simulink model "r2_deng_tvg_rev1_13"  (R2012b)
settings: Solver=VariableStepDiscrete  StartTime=0.0  StopTime=2000  RelTol=1e-3
libraries: xbsIndex_r4 x7993, casper_library_misc x17, casper_library_sources x12, casper_library_communications x4, simulink x3, xps_library x2
(part 9 of 65)

== system r2_deng_tvg_rev1_13/bus_expand3 ==
  bus_in : Inport
  gatewayOut{1..8} (8 alike) : xbsIndex_r4/Gateway Out  inherit_from_input=off  hdl_port=off  timing_constraint=None  locs_specified=off  LOCs={}  UseAsDAC=off  DACChannel='1'  block_type=gatewayout
  reinterpret{1..8} (8 alike) : xbsIndex_r4/Reinterpret  force_arith_type=on  arith_type="Signed  (2's comp)"  force_bin_pt=on  bin_pt=19  block_type=reinterpret
  slice1 : xbsIndex_r4/Slice  nbits=20  boolean_output=off  mode=Upper Bit Location + Width  bit1=-140  base1=MSB of Input  bit0=0  base0=LSB of Input  dbl_ovrd=off  block_type=slice
  slice2 : xbsIndex_r4/Slice  nbits=20  boolean_output=off  mode=Upper Bit Location + Width  bit1=-120  base1=MSB of Input  bit0=0  base0=LSB of Input  dbl_ovrd=off  block_type=slice
  slice3 : xbsIndex_r4/Slice  nbits=20  boolean_output=off  mode=Upper Bit Location + Width  bit1=-100  base1=MSB of Input  bit0=0  base0=LSB of Input  dbl_ovrd=off  block_type=slice
  slice4 : xbsIndex_r4/Slice  nbits=20  boolean_output=off  mode=Upper Bit Location + Width  bit1=-80  base1=MSB of Input  bit0=0  base0=LSB of Input  dbl_ovrd=off  block_type=slice
  slice5 : xbsIndex_r4/Slice  nbits=20  boolean_output=off  mode=Upper Bit Location + Width  bit1=-60  base1=MSB of Input  bit0=0  base0=LSB of Input  dbl_ovrd=off  block_type=slice
  slice6 : xbsIndex_r4/Slice  nbits=20  boolean_output=off  mode=Upper Bit Location + Width  bit1=-40  base1=MSB of Input  bit0=0  base0=LSB of Input  dbl_ovrd=off  block_type=slice
  slice7 : xbsIndex_r4/Slice  nbits=20  boolean_output=off  mode=Upper Bit Location + Width  bit1=-20  base1=MSB of Input  bit0=0  base0=LSB of Input  dbl_ovrd=off  block_type=slice
  slice8 : xbsIndex_r4/Slice  nbits=20  boolean_output=off  mode=Upper Bit Location + Width  bit1=0  base1=MSB of Input  bit0=0  base0=LSB of Input  dbl_ovrd=off  block_type=slice
  toWorkspace1 : ToWorkspace  VariableName=wng0_tp0_1  SampleTime=-1  SaveFormat=Structure With Time
  toWorkspace2 : ToWorkspace  VariableName=wng0_tp0_2  SampleTime=-1  SaveFormat=Structure With Time
  toWorkspace3 : ToWorkspace  VariableName=wng0_tp0_3  SampleTime=-1  SaveFormat=Structure With Time
  toWorkspace4 : ToWorkspace  VariableName=wng0_tp0_4  SampleTime=-1  SaveFormat=Structure With Time
  toWorkspace5 : ToWorkspace  VariableName=wng0_tp0_5  SampleTime=-1  SaveFormat=Structure With Time
  toWorkspace6 : ToWorkspace  VariableName=wng0_tp0_6  SampleTime=-1  SaveFormat=Structure With Time
  toWorkspace7 : ToWorkspace  VariableName=wng0_tp0_7  SampleTime=-1  SaveFormat=Structure With Time
  toWorkspace8 : ToWorkspace  VariableName=wng0_tp0_8  SampleTime=-1  SaveFormat=Structure With Time
  msb_out8 : Outport
  out7 : Outport  Port=2
  out6 : Outport  Port=3
  out5 : Outport  Port=4
  out4 : Outport  Port=5
  out3 : Outport  Port=6
  out2 : Outport  Port=7
  lsb_out1 : Outport  Port=8
  wires:
  bus_in/1 -> slice8/1, slice7/1, slice6/1, slice5/1, slice4/1, slice3/1, slice2/1, slice1/1
  slice8/1 -> reinterpret8/1
  reinterpret8/1 -> gatewayOut8/1, msb_out8/1
  gatewayOut8/1 -> toWorkspace8/1
  slice7/1 -> reinterpret7/1
  reinterpret7/1 -> gatewayOut7/1, out7/1
  gatewayOut7/1 -> toWorkspace7/1
  slice6/1 -> reinterpret6/1
  reinterpret6/1 -> gatewayOut6/1, out6/1
  gatewayOut6/1 -> toWorkspace6/1
  slice5/1 -> reinterpret5/1
  reinterpret5/1 -> gatewayOut5/1, out5/1
  gatewayOut5/1 -> toWorkspace5/1
  slice4/1 -> reinterpret4/1
  reinterpret4/1 -> gatewayOut4/1, out4/1
  gatewayOut4/1 -> toWorkspace4/1
  slice3/1 -> reinterpret3/1
  reinterpret3/1 -> gatewayOut3/1, out3/1
  gatewayOut3/1 -> toWorkspace3/1
  slice2/1 -> reinterpret2/1
  reinterpret2/1 -> gatewayOut2/1, out2/1
  gatewayOut2/1 -> toWorkspace2/1
  slice1/1 -> reinterpret1/1
  reinterpret1/1 -> gatewayOut1/1, lsb_out1/1
  gatewayOut1/1 -> toWorkspace1/1

== system r2_deng_tvg_rev1_13/bus_expand4 ==
  bus_in : Inport
  gatewayOut{1..8} (8 alike) : xbsIndex_r4/Gateway Out  inherit_from_input=off  hdl_port=off  timing_constraint=None  locs_specified=off  LOCs={}  UseAsDAC=off  DACChannel='1'  block_type=gatewayout
  reinterpret{1..8} (8 alike) : xbsIndex_r4/Reinterpret  force_arith_type=on  arith_type="Signed  (2's comp)"  force_bin_pt=on  bin_pt=17  block_type=reinterpret
  slice1 : xbsIndex_r4/Slice  nbits=18  boolean_output=off  mode=Upper Bit Location + Width  bit1=-126  base1=MSB of Input  bit0=0  base0=LSB of Input  dbl_ovrd=off  block_type=slice
  slice2 : xbsIndex_r4/Slice  nbits=18  boolean_output=off  mode=Upper Bit Location + Width  bit1=-108  base1=MSB of Input  bit0=0  base0=LSB of Input  dbl_ovrd=off  block_type=slice
  slice3 : xbsIndex_r4/Slice  nbits=18  boolean_output=off  mode=Upper Bit Location + Width  bit1=-90  base1=MSB of Input  bit0=0  base0=LSB of Input  dbl_ovrd=off  block_type=slice
  slice4 : xbsIndex_r4/Slice  nbits=18  boolean_output=off  mode=Upper Bit Location + Width  bit1=-72  base1=MSB of Input  bit0=0  base0=LSB of Input  dbl_ovrd=off  block_type=slice
  slice5 : xbsIndex_r4/Slice  nbits=18  boolean_output=off  mode=Upper Bit Location + Width  bit1=-54  base1=MSB of Input  bit0=0  base0=LSB of Input  dbl_ovrd=off  block_type=slice
  slice6 : xbsIndex_r4/Slice  nbits=18  boolean_output=off  mode=Upper Bit Location + Width  bit1=-36  base1=MSB of Input  bit0=0  base0=LSB of Input  dbl_ovrd=off  block_type=slice
  slice7 : xbsIndex_r4/Slice  nbits=18  boolean_output=off  mode=Upper Bit Location + Width  bit1=-18  base1=MSB of Input  bit0=0  base0=LSB of Input  dbl_ovrd=off  block_type=slice
  slice8 : xbsIndex_r4/Slice  nbits=18  boolean_output=off  mode=Upper Bit Location + Width  bit1=0  base1=MSB of Input  bit0=0  base0=LSB of Input  dbl_ovrd=off  block_type=slice
  toWorkspace1 : ToWorkspace  VariableName=cwg1_tp0_1  SampleTime=-1  SaveFormat=Structure With Time
  toWorkspace2 : ToWorkspace  VariableName=cwg1_tp0_2  SampleTime=-1  SaveFormat=Structure With Time
  toWorkspace3 : ToWorkspace  VariableName=cwg1_tp0_3  SampleTime=-1  SaveFormat=Structure With Time
  toWorkspace4 : ToWorkspace  VariableName=cwg1_tp0_4  SampleTime=-1  SaveFormat=Structure With Time
  toWorkspace5 : ToWorkspace  VariableName=cwg1_tp0_5  SampleTime=-1  SaveFormat=Structure With Time
  toWorkspace6 : ToWorkspace  VariableName=cwg1_tp0_6  SampleTime=-1  SaveFormat=Structure With Time
  toWorkspace7 : ToWorkspace  VariableName=cwg1_tp0_7  SampleTime=-1  SaveFormat=Structure With Time
  toWorkspace8 : ToWorkspace  VariableName=cwg1_tp0_8  SampleTime=-1  SaveFormat=Structure With Time
  msb_out8 : Outport
  out7 : Outport  Port=2
  out6 : Outport  Port=3
  out5 : Outport  Port=4
  out4 : Outport  Port=5
  out3 : Outport  Port=6
  out2 : Outport  Port=7
  lsb_out1 : Outport  Port=8
  wires:
  bus_in/1 -> slice8/1, slice7/1, slice6/1, slice5/1, slice4/1, slice3/1, slice2/1, slice1/1
  slice8/1 -> reinterpret8/1
  reinterpret8/1 -> gatewayOut8/1, msb_out8/1
  gatewayOut8/1 -> toWorkspace8/1
  slice7/1 -> reinterpret7/1
  reinterpret7/1 -> gatewayOut7/1, out7/1
  gatewayOut7/1 -> toWorkspace7/1
  slice6/1 -> reinterpret6/1
  reinterpret6/1 -> gatewayOut6/1, out6/1
  gatewayOut6/1 -> toWorkspace6/1
  slice5/1 -> reinterpret5/1
  reinterpret5/1 -> gatewayOut5/1, out5/1
  gatewayOut5/1 -> toWorkspace5/1
  slice4/1 -> reinterpret4/1
  reinterpret4/1 -> gatewayOut4/1, out4/1
  gatewayOut4/1 -> toWorkspace4/1
  slice3/1 -> reinterpret3/1
  reinterpret3/1 -> gatewayOut3/1, out3/1
  gatewayOut3/1 -> toWorkspace3/1
  slice2/1 -> reinterpret2/1
  reinterpret2/1 -> gatewayOut2/1, out2/1
  gatewayOut2/1 -> toWorkspace2/1
  slice1/1 -> reinterpret1/1
  reinterpret1/1 -> gatewayOut1/1, lsb_out1/1
  gatewayOut1/1 -> toWorkspace1/1

== system r2_deng_tvg_rev1_13/bus_expand6 ==
  bus_in : Inport
  gatewayOut{1..8} (8 alike) : xbsIndex_r4/Gateway Out  inherit_from_input=off  hdl_port=off  timing_constraint=None  locs_specified=off  LOCs={}  UseAsDAC=off  DACChannel='1'  block_type=gatewayout
  reinterpret{1..8} (8 alike) : xbsIndex_r4/Reinterpret  force_arith_type=on  arith_type="Signed  (2's comp)"  force_bin_pt=on  bin_pt=9  block_type=reinterpret
  slice1 : xbsIndex_r4/Slice  nbits=10  boolean_output=off  mode=Upper Bit Location + Width  bit1=-70  base1=MSB of Input  bit0=0  base0=LSB of Input  dbl_ovrd=off  block_type=slice
  slice2 : xbsIndex_r4/Slice  nbits=10  boolean_output=off  mode=Upper Bit Location + Width  bit1=-60  base1=MSB of Input  bit0=0  base0=LSB of Input  dbl_ovrd=off  block_type=slice
  slice3 : xbsIndex_r4/Slice  nbits=10  boolean_output=off  mode=Upper Bit Location + Width  bit1=-50  base1=MSB of Input  bit0=0  base0=LSB of Input  dbl_ovrd=off  block_type=slice
  slice4 : xbsIndex_r4/Slice  nbits=10  boolean_output=off  mode=Upper Bit Location + Width  bit1=-40  base1=MSB of Input  bit0=0  base0=LSB of Input  dbl_ovrd=off  block_type=slice
  slice5 : xbsIndex_r4/Slice  nbits=10  boolean_output=off  mode=Upper Bit Location + Width  bit1=-30  base1=MSB of Input  bit0=0  base0=LSB of Input  dbl_ovrd=off  block_type=slice
  slice6 : xbsIndex_r4/Slice  nbits=10  boolean_output=off  mode=Upper Bit Location + Width  bit1=-20  base1=MSB of Input  bit0=0  base0=LSB of Input  dbl_ovrd=off  block_type=slice
  slice7 : xbsIndex_r4/Slice  nbits=10  boolean_output=off  mode=Upper Bit Location + Width  bit1=-10  base1=MSB of Input  bit0=0  base0=LSB of Input  dbl_ovrd=off  block_type=slice
  slice8 : xbsIndex_r4/Slice  nbits=10  boolean_output=off  mode=Upper Bit Location + Width  bit1=0  base1=MSB of Input  bit0=0  base0=LSB of Input  dbl_ovrd=off  block_type=slice
  toWorkspace1 : ToWorkspace  VariableName=cwg1_tp2_1  SampleTime=-1  SaveFormat=Structure With Time
  toWorkspace2 : ToWorkspace  VariableName=cwg1_tp2_2  SampleTime=-1  SaveFormat=Structure With Time
  toWorkspace3 : ToWorkspace  VariableName=cwg1_tp2_3  SampleTime=-1  SaveFormat=Structure With Time
  toWorkspace4 : ToWorkspace  VariableName=cwg1_tp2_4  SampleTime=-1  SaveFormat=Structure With Time
  toWorkspace5 : ToWorkspace  VariableName=cwg1_tp2_5  SampleTime=-1  SaveFormat=Structure With Time
  toWorkspace6 : ToWorkspace  VariableName=cwg1_tp2_6  SampleTime=-1  SaveFormat=Structure With Time
  toWorkspace7 : ToWorkspace  VariableName=cwg1_tp2_7  SampleTime=-1  SaveFormat=Structure With Time
  toWorkspace8 : ToWorkspace  VariableName=cwg1_tp2_8  SampleTime=-1  SaveFormat=Structure With Time
  msb_out8 : Outport
  out7 : Outport  Port=2
  out6 : Outport  Port=3
  out5 : Outport  Port=4
  out4 : Outport  Port=5
  out3 : Outport  Port=6
  out2 : Outport  Port=7
  lsb_out1 : Outport  Port=8
  wires:
  bus_in/1 -> slice8/1, slice7/1, slice6/1, slice5/1, slice4/1, slice3/1, slice2/1, slice1/1
  slice8/1 -> reinterpret8/1
  reinterpret8/1 -> gatewayOut8/1, msb_out8/1
  gatewayOut8/1 -> toWorkspace8/1
  slice7/1 -> reinterpret7/1
  reinterpret7/1 -> gatewayOut7/1, out7/1
  gatewayOut7/1 -> toWorkspace7/1
  slice6/1 -> reinterpret6/1
  reinterpret6/1 -> gatewayOut6/1, out6/1
  gatewayOut6/1 -> toWorkspace6/1
  slice5/1 -> reinterpret5/1
  reinterpret5/1 -> gatewayOut5/1, out5/1
  gatewayOut5/1 -> toWorkspace5/1
  slice4/1 -> reinterpret4/1
  reinterpret4/1 -> gatewayOut4/1, out4/1
  gatewayOut4/1 -> toWorkspace4/1
  slice3/1 -> reinterpret3/1
  reinterpret3/1 -> gatewayOut3/1, out3/1
  gatewayOut3/1 -> toWorkspace3/1
  slice2/1 -> reinterpret2/1
  reinterpret2/1 -> gatewayOut2/1, out2/1
  gatewayOut2/1 -> toWorkspace2/1
  slice1/1 -> reinterpret1/1
  reinterpret1/1 -> gatewayOut1/1, lsb_out1/1
  gatewayOut1/1 -> toWorkspace1/1

== system r2_deng_tvg_rev1_13/bus_expand8 ==
  bus_in : Inport
  gatewayOut{1..8} (8 alike) : xbsIndex_r4/Gateway Out  inherit_from_input=off  hdl_port=off  timing_constraint=None  locs_specified=off  LOCs={}  UseAsDAC=off  DACChannel='1'  block_type=gatewayout
  reinterpret{1..8} (8 alike) : xbsIndex_r4/Reinterpret  force_arith_type=on  arith_type="Signed  (2's comp)"  force_bin_pt=on  bin_pt=17  block_type=reinterpret
  slice1 : xbsIndex_r4/Slice  nbits=18  boolean_output=off  mode=Upper Bit Location + Width  bit1=-126  base1=MSB of Input  bit0=0  base0=LSB of Input  dbl_ovrd=off  block_type=slice
  slice2 : xbsIndex_r4/Slice  nbits=18  boolean_output=off  mode=Upper Bit Location + Width  bit1=-108  base1=MSB of Input  bit0=0  base0=LSB of Input  dbl_ovrd=off  block_type=slice
  slice3 : xbsIndex_r4/Slice  nbits=18  boolean_output=off  mode=Upper Bit Location + Width  bit1=-90  base1=MSB of Input  bit0=0  base0=LSB of Input  dbl_ovrd=off  block_type=slice
  slice4 : xbsIndex_r4/Slice  nbits=18  boolean_output=off  mode=Upper Bit Location + Width  bit1=-72  base1=MSB of Input  bit0=0  base0=LSB of Input  dbl_ovrd=off  block_type=slice
  slice5 : xbsIndex_r4/Slice  nbits=18  boolean_output=off  mode=Upper Bit Location + Width  bit1=-54  base1=MSB of Input  bit0=0  base0=LSB of Input  dbl_ovrd=off  block_type=slice
  slice6 : xbsIndex_r4/Slice  nbits=18  boolean_output=off  mode=Upper Bit Location + Width  bit1=-36  base1=MSB of Input  bit0=0  base0=LSB of Input  dbl_ovrd=off  block_type=slice
  slice7 : xbsIndex_r4/Slice  nbits=18  boolean_output=off  mode=Upper Bit Location + Width  bit1=-18  base1=MSB of Input  bit0=0  base0=LSB of Input  dbl_ovrd=off  block_type=slice
  slice8 : xbsIndex_r4/Slice  nbits=18  boolean_output=off  mode=Upper Bit Location + Width  bit1=0  base1=MSB of Input  bit0=0  base0=LSB of Input  dbl_ovrd=off  block_type=slice
  toWorkspace1 : ToWorkspace  VariableName=wng1_tp0_1  SampleTime=-1  SaveFormat=Structure With Time
  toWorkspace2 : ToWorkspace  VariableName=wng1_tp0_2  SampleTime=-1  SaveFormat=Structure With Time
  toWorkspace3 : ToWorkspace  VariableName=wng1_tp0_3  SampleTime=-1  SaveFormat=Structure With Time
  toWorkspace4 : ToWorkspace  VariableName=wng1_tp0_4  SampleTime=-1  SaveFormat=Structure With Time
  toWorkspace5 : ToWorkspace  VariableName=wng1_tp0_5  SampleTime=-1  SaveFormat=Structure With Time
  toWorkspace6 : ToWorkspace  VariableName=wng1_tp0_6  SampleTime=-1  SaveFormat=Structure With Time
  toWorkspace7 : ToWorkspace  VariableName=wng1_tp0_7  SampleTime=-1  SaveFormat=Structure With Time
  toWorkspace8 : ToWorkspace  VariableName=wng1_tp0_8  SampleTime=-1  SaveFormat=Structure With Time
  msb_out8 : Outport
  out7 : Outport  Port=2
  out6 : Outport  Port=3
  out5 : Outport  Port=4
  out4 : Outport  Port=5
  out3 : Outport  Port=6
  out2 : Outport  Port=7
  lsb_out1 : Outport  Port=8
  wires:
  bus_in/1 -> slice8/1, slice7/1, slice6/1, slice5/1, slice4/1, slice3/1, slice2/1, slice1/1
  slice8/1 -> reinterpret8/1
  reinterpret8/1 -> gatewayOut8/1, msb_out8/1
  gatewayOut8/1 -> toWorkspace8/1
  slice7/1 -> reinterpret7/1
  reinterpret7/1 -> gatewayOut7/1, out7/1
  gatewayOut7/1 -> toWorkspace7/1
  slice6/1 -> reinterpret6/1
  reinterpret6/1 -> gatewayOut6/1, out6/1
  gatewayOut6/1 -> toWorkspace6/1
  slice5/1 -> reinterpret5/1
  reinterpret5/1 -> gatewayOut5/1, out5/1
  gatewayOut5/1 -> toWorkspace5/1
  slice4/1 -> reinterpret4/1
  reinterpret4/1 -> gatewayOut4/1, out4/1
  gatewayOut4/1 -> toWorkspace4/1
  slice3/1 -> reinterpret3/1
  reinterpret3/1 -> gatewayOut3/1, out3/1
  gatewayOut3/1 -> toWorkspace3/1
  slice2/1 -> reinterpret2/1
  reinterpret2/1 -> gatewayOut2/1, out2/1
  gatewayOut2/1 -> toWorkspace2/1
  slice1/1 -> reinterpret1/1
  reinterpret1/1 -> gatewayOut1/1, lsb_out1/1
  gatewayOut1/1 -> toWorkspace1/1

== system r2_deng_tvg_rev1_13/bus_expand9 ==
  bus_in : Inport
  gatewayOut{1..8} (8 alike) : xbsIndex_r4/Gateway Out  inherit_from_input=off  hdl_port=off  timing_constraint=None  locs_specified=off  LOCs={}  UseAsDAC=off  DACChannel='1'  block_type=gatewayout
  reinterpret{1..8} (8 alike) : xbsIndex_r4/Reinterpret  force_arith_type=on  arith_type=Unsigned  force_bin_pt=on  bin_pt=0  block_type=reinterpret
  slice1 : xbsIndex_r4/Slice  nbits=10  boolean_output=off  mode=Upper Bit Location + Width  bit1=-70  base1=MSB of Input  bit0=0  base0=LSB of Input  dbl_ovrd=off  block_type=slice
  slice2 : xbsIndex_r4/Slice  nbits=10  boolean_output=off  mode=Upper Bit Location + Width  bit1=-60  base1=MSB of Input  bit0=0  base0=LSB of Input  dbl_ovrd=off  block_type=slice
  slice3 : xbsIndex_r4/Slice  nbits=10  boolean_output=off  mode=Upper Bit Location + Width  bit1=-50  base1=MSB of Input  bit0=0  base0=LSB of Input  dbl_ovrd=off  block_type=slice
  slice4 : xbsIndex_r4/Slice  nbits=10  boolean_output=off  mode=Upper Bit Location + Width  bit1=-40  base1=MSB of Input  bit0=0  base0=LSB of Input  dbl_ovrd=off  block_type=slice
  slice5 : xbsIndex_r4/Slice  nbits=10  boolean_output=off  mode=Upper Bit Location + Width  bit1=-30  base1=MSB of Input  bit0=0  base0=LSB of Input  dbl_ovrd=off  block_type=slice
  slice6 : xbsIndex_r4/Slice  nbits=10  boolean_output=off  mode=Upper Bit Location + Width  bit1=-20  base1=MSB of Input  bit0=0  base0=LSB of Input  dbl_ovrd=off  block_type=slice
  slice7 : xbsIndex_r4/Slice  nbits=10  boolean_output=off  mode=Upper Bit Location + Width  bit1=-10  base1=MSB of Input  bit0=0  base0=LSB of Input  dbl_ovrd=off  block_type=slice
  slice8 : xbsIndex_r4/Slice  nbits=10  boolean_output=off  mode=Upper Bit Location + Width  bit1=0  base1=MSB of Input  bit0=0  base0=LSB of Input  dbl_ovrd=off  block_type=slice
  toWorkspace1 : ToWorkspace  VariableName=Data_Mux1_1  SampleTime=-1  SaveFormat=Structure With Time
  toWorkspace2 : ToWorkspace  VariableName=Data_Mux1_2  SampleTime=-1  SaveFormat=Structure With Time
  toWorkspace3 : ToWorkspace  VariableName=Data_Mux1_3  SampleTime=-1  SaveFormat=Structure With Time
  toWorkspace4 : ToWorkspace  VariableName=Data_Mux1_4  SampleTime=-1  SaveFormat=Structure With Time
  toWorkspace5 : ToWorkspace  VariableName=Data_Mux1_5  SampleTime=-1  SaveFormat=Structure With Time
  toWorkspace6 : ToWorkspace  VariableName=Data_Mux1_6  SampleTime=-1  SaveFormat=Structure With Time
  toWorkspace7 : ToWorkspace  VariableName=Data_Mux1_7  SampleTime=-1  SaveFormat=Structure With Time
  toWorkspace8 : ToWorkspace  VariableName=Data_Mux1_8  SampleTime=-1  SaveFormat=Structure With Time
  msb_out8 : Outport
  out7 : Outport  Port=2
  out6 : Outport  Port=3
  out5 : Outport  Port=4
  out4 : Outport  Port=5
  out3 : Outport  Port=6
  out2 : Outport  Port=7
  lsb_out1 : Outport  Port=8
  wires:
  bus_in/1 -> slice8/1, slice7/1, slice6/1, slice5/1, slice4/1, slice3/1, slice2/1, slice1/1
  slice8/1 -> reinterpret8/1
  reinterpret8/1 -> gatewayOut8/1, msb_out8/1
  gatewayOut8/1 -> toWorkspace8/1
  slice7/1 -> reinterpret7/1
  reinterpret7/1 -> gatewayOut7/1, out7/1
  gatewayOut7/1 -> toWorkspace7/1
  slice6/1 -> reinterpret6/1
  reinterpret6/1 -> gatewayOut6/1, out6/1
  gatewayOut6/1 -> toWorkspace6/1
  slice5/1 -> reinterpret5/1
  reinterpret5/1 -> gatewayOut5/1, out5/1
  gatewayOut5/1 -> toWorkspace5/1
  slice4/1 -> reinterpret4/1
  reinterpret4/1 -> gatewayOut4/1, out4/1
  gatewayOut4/1 -> toWorkspace4/1
  slice3/1 -> reinterpret3/1
  reinterpret3/1 -> gatewayOut3/1, out3/1
  gatewayOut3/1 -> toWorkspace3/1
  slice2/1 -> reinterpret2/1
  reinterpret2/1 -> gatewayOut2/1, out2/1
  gatewayOut2/1 -> toWorkspace2/1
  slice1/1 -> reinterpret1/1
  reinterpret1/1 -> gatewayOut1/1, lsb_out1/1
  gatewayOut1/1 -> toWorkspace1/1

== system r2_deng_tvg_rev1_13/bus_mult ==
  a : Inport
  b : Inport  Port=2
  a*b_bussify : Subsystem  AncestorBlock=casper_library_flow_control/bus_create  mask(bus_create){inputNum=8}
      mask prompts: inputNum "Number of inputs:"
      mask init:
      | bus_create_init(gcb,...
      |     'inputNum', inputNum);
  a_debus : Subsystem  AncestorBlock=casper_library_flow_control/bus_expand  mask(bus_expand){mode=divisions of arbitrary size, outputNum=1, outputWidth=[38 38 38 38 38 38 38 38], outputBinaryPt=[34 34 34 34 34 34 34 34], outputArithmeticType=[1 1 1 1 1 1 1 1], show_format=on, outputToWorkspace=off, variablePrefix=, outputToModelAsWell=on}
      mask prompts: outputNum "Number of outputs:"; outputWidth "Output width [msb ... lsb]:"; outputBinaryPt "Output binary point position [msb ... lsb]:"; outputArithmeticType "Output arithmetic type (ufix=0, fix=1, bool=2) [msb ... lsb]:"; show_format "Print format string?"; outputToWorkspace "Output to workspace?"; variablePrefix "Variable name prefix:"; outputToModelAsWell "Output to model as well?"
      mask help:
      | Expands a 'bus' made using a bus_create or Xilinx
      | concat block.
      | The input will be divided into the specified number
      | of outputs with the specified arithmetic types.
      | Divisions are made from most significant bit.
      mask init: same as r2_deng_tvg_rev1_13/bus_expand
      settings: AttributesFormatString=8 outputs: f38.34,f38.34,f38.34,f38.34,f38.34,f38.34,f38.34,f38.34,
      mask TypeOptions mode: divisions of equal size | divisions of arbitrary size
      mask Callback mode: bus_expand_callback();
      mask Callback outputWidth: bus_expand_callback();
      mask Callback outputToWorkspace: bus_expand_callback();
  b_debus : Subsystem  AncestorBlock=casper_library_flow_control/bus_expand  mask(bus_expand){mode=divisions of arbitrary size, outputNum=1, outputWidth=[16 16 16 16 16 16 16 16], outputBinaryPt=[15 15 15 15 15 15 15 15], outputArithmeticType=[0 0 0 0 0 0 0 0], show_format=on, outputToWorkspace=off, variablePrefix=, outputToModelAsWell=on}
      mask prompts: outputNum "Number of outputs:"; outputWidth "Output width [msb ... lsb]:"; outputBinaryPt "Output binary point position [msb ... lsb]:"; outputArithmeticType "Output arithmetic type (ufix=0, fix=1, bool=2) [msb ... lsb]:"; show_format "Print format string?"; outputToWorkspace "Output to workspace?"; variablePrefix "Variable name prefix:"; outputToModelAsWell "Output to model as well?"
      mask help:
      | Expands a 'bus' made using a bus_create or Xilinx
      | concat block.
      | The input will be divided into the specified number
      | of outputs with the specified arithmetic types.
      | Divisions are made from most significant bit.
      mask init: same as r2_deng_tvg_rev1_13/bus_expand
      settings: AttributesFormatString=8 outputs: uf16.15,uf16.15,uf16.15,uf16.15,uf16.15,uf16.15,uf16.15,uf16.15,
      mask TypeOptions mode: divisions of equal size | divisions of arbitrary size
      mask Callback mode: bus_expand_callback();
      mask Callback outputWidth: bus_expand_callback();
      mask Callback outputToWorkspace: bus_expand_callback();
  mult{1..8} (8 alike) : xbsIndex_r4/Mult  precision=User Defined  arith_type="Signed  (2's comp)"  n_bits=54  bin_pt=49  quantization="Round  (unbiased: +/- Inf)"  overflow=Saturate  en=off  latency=mult_latency  dbl_ovrd=off  use_behavioral_HDL=on  opt=Speed  use_embedded=off  optimum_pipeline=off  pipeline=on  use_rpm=on  placement_style=Triangular  block_type=mult
  repa : Subsystem  AncestorBlock=casper_library_bus/bus_replicate  mask(bus_replicate){replication=1, latency=3, misc=off, implementation=core}
      mask prompts: replication "replication factor"; misc "misc support"; implementation "delay implementation"
      mask help: Output bus formed by replicating input bus a number of times
      mask init:
      | bus_replicate_init(gcb, ...
      |     'replication', replication, ...
      |     'latency', latency, ...
      |     'implementation', implementation, ...
      |     'misc', misc);
      mask TypeOptions implementation: core | behavioral
  repb : Subsystem  AncestorBlock=casper_library_bus/bus_replicate  mask(bus_replicate){replication=8, latency=3, misc=off, implementation=core}
      mask prompts: replication "replication factor"; misc "misc support"; implementation "delay implementation"
      mask help: Output bus formed by replicating input bus a number of times
      mask init:
      | bus_replicate_init(gcb, ...
      |     'replication', replication, ...
      |     'latency', latency, ...
      |     'implementation', implementation, ...
      |     'misc', misc);
      mask TypeOptions implementation: core | behavioral
  a*b : Outport
  wires:
  a/1 -> repa/1(in)
  b/1 -> repb/1(in)
  repa/1(out) -> a_debus/1(bus_in)
  repb/1(out) -> b_debus/1(bus_in)
  a_debus/1(msb_out8) -> mult1/1
  b_debus/1(msb_out8) -> mult1/2
  a_debus/2(out7) -> mult2/1
  b_debus/2(out7) -> mult2/2
  a_debus/3(out6) -> mult3/1
  b_debus/3(out6) -> mult3/2
  a_debus/4(out5) -> mult4/1
  b_debus/4(out5) -> mult4/2
  a_debus/5(out4) -> mult5/1
  b_debus/5(out4) -> mult5/2
  a_debus/6(out3) -> mult6/1
  b_debus/6(out3) -> mult6/2
  a_debus/7(out2) -> mult7/1
  b_debus/7(out2) -> mult7/2
  a_debus/8(lsb_out1) -> mult8/1
  b_debus/8(lsb_out1) -> mult8/2
  mult1/1 -> a*b_bussify/1(in1)
  mult2/1 -> a*b_bussify/2(in2)
  mult3/1 -> a*b_bussify/3(in3)
  mult4/1 -> a*b_bussify/4(in4)
  mult5/1 -> a*b_bussify/5(in5)
  mult6/1 -> a*b_bussify/6(in6)
  mult7/1 -> a*b_bussify/7(in7)
  mult8/1 -> a*b_bussify/8(in8)
  a*b_bussify/1(bus_out) -> a*b/1

== system r2_deng_tvg_rev1_13/bus_mult1 ==
  a : Inport
  b : Inport  Port=2
  a*b_bussify : Subsystem  AncestorBlock=casper_library_flow_control/bus_create  mask(bus_create){inputNum=8}
      mask prompts: inputNum "Number of inputs:"
      mask init:
      | bus_create_init(gcb,...
      |     'inputNum', inputNum);
  a_debus : Subsystem  AncestorBlock=casper_library_flow_control/bus_expand  mask(bus_expand){mode=divisions of arbitrary size, outputNum=1, outputWidth=[38 38 38 38 38 38 38 38], outputBinaryPt=[34 34 34 34 34 34 34 34], outputArithmeticType=[1 1 1 1 1 1 1 1], show_format=on, outputToWorkspace=off, variablePrefix=, outputToModelAsWell=on}
      mask prompts: outputNum "Number of outputs:"; outputWidth "Output width [msb ... lsb]:"; outputBinaryPt "Output binary point position [msb ... lsb]:"; outputArithmeticType "Output arithmetic type (ufix=0, fix=1, bool=2) [msb ... lsb]:"; show_format "Print format string?"; outputToWorkspace "Output to workspace?"; variablePrefix "Variable name prefix:"; outputToModelAsWell "Output to model as well?"
      mask help:
      | Expands a 'bus' made using a bus_create or Xilinx
      | concat block.
      | The input will be divided into the specified number
      | of outputs with the specified arithmetic types.
      | Divisions are made from most significant bit.
      mask init: same as r2_deng_tvg_rev1_13/bus_expand
      settings: AttributesFormatString=8 outputs: f38.34,f38.34,f38.34,f38.34,f38.34,f38.34,f38.34,f38.34,
      mask TypeOptions mode: divisions of equal size | divisions of arbitrary size
      mask Callback mode: bus_expand_callback();
      mask Callback outputWidth: bus_expand_callback();
      mask Callback outputToWorkspace: bus_expand_callback();
  b_debus : Subsystem  AncestorBlock=casper_library_flow_control/bus_expand  mask(bus_expand){mode=divisions of arbitrary size, outputNum=1, outputWidth=[16 16 16 16 16 16 16 16], outputBinaryPt=[15 15 15 15 15 15 15 15], outputArithmeticType=[0 0 0 0 0 0 0 0], show_format=on, outputToWorkspace=off, variablePrefix=, outputToModelAsWell=on}
      mask prompts: outputNum "Number of outputs:"; outputWidth "Output width [msb ... lsb]:"; outputBinaryPt "Output binary point position [msb ... lsb]:"; outputArithmeticType "Output arithmetic type (ufix=0, fix=1, bool=2) [msb ... lsb]:"; show_format "Print format string?"; outputToWorkspace "Output to workspace?"; variablePrefix "Variable name prefix:"; outputToModelAsWell "Output to model as well?"
      mask help:
      | Expands a 'bus' made using a bus_create or Xilinx
      | concat block.
      | The input will be divided into the specified number
      | of outputs with the specified arithmetic types.
      | Divisions are made from most significant bit.
      mask init: same as r2_deng_tvg_rev1_13/bus_expand
      settings: AttributesFormatString=8 outputs: uf16.15,uf16.15,uf16.15,uf16.15,uf16.15,uf16.15,uf16.15,uf16.15,
      mask TypeOptions mode: divisions of equal size | divisions of arbitrary size
      mask Callback mode: bus_expand_callback();
      mask Callback outputWidth: bus_expand_callback();
      mask Callback outputToWorkspace: bus_expand_callback();
  mult{1..8} (8 alike) : xbsIndex_r4/Mult  precision=User Defined  arith_type="Signed  (2's comp)"  n_bits=54  bin_pt=49  quantization="Round  (unbiased: +/- Inf)"  overflow=Saturate  en=off  latency=mult_latency  dbl_ovrd=off  use_behavioral_HDL=on  opt=Speed  use_embedded=off  optimum_pipeline=off  pipeline=on  use_rpm=on  placement_style=Triangular  block_type=mult
  repa : Subsystem  AncestorBlock=casper_library_bus/bus_replicate  mask(bus_replicate){replication=1, latency=3, misc=off, implementation=core}
      mask prompts: replication "replication factor"; misc "misc support"; implementation "delay implementation"
      mask help: Output bus formed by replicating input bus a number of times
      mask init:
      | bus_replicate_init(gcb, ...
      |     'replication', replication, ...
      |     'latency', latency, ...
      |     'implementation', implementation, ...
      |     'misc', misc);
      mask TypeOptions implementation: core | behavioral
  repb : Subsystem  AncestorBlock=casper_library_bus/bus_replicate  mask(bus_replicate){replication=8, latency=3, misc=off, implementation=core}
      mask prompts: replication "replication factor"; misc "misc support"; implementation "delay implementation"
      mask help: Output bus formed by replicating input bus a number of times
      mask init:
      | bus_replicate_init(gcb, ...
      |     'replication', replication, ...
      |     'latency', latency, ...
      |     'implementation', implementation, ...
      |     'misc', misc);
      mask TypeOptions implementation: core | behavioral
  a*b : Outport
  wires:
  a*b_bussify/1(bus_out) -> a*b/1
  mult8/1 -> a*b_bussify/8(in8)
  mult7/1 -> a*b_bussify/7(in7)
  mult6/1 -> a*b_bussify/6(in6)
  mult5/1 -> a*b_bussify/5(in5)
  mult4/1 -> a*b_bussify/4(in4)
  mult3/1 -> a*b_bussify/3(in3)
  mult2/1 -> a*b_bussify/2(in2)
  mult1/1 -> a*b_bussify/1(in1)
  b_debus/8(lsb_out1) -> mult8/2
  a_debus/8(lsb_out1) -> mult8/1
  b_debus/7(out2) -> mult7/2
  a_debus/7(out2) -> mult7/1
  b_debus/6(out3) -> mult6/2
  a_debus/6(out3) -> mult6/1
  b_debus/5(out4) -> mult5/2
  a_debus/5(out4) -> mult5/1
  b_debus/4(out5) -> mult4/2
  a_debus/4(out5) -> mult4/1
  b_debus/3(out6) -> mult3/2
  a_debus/3(out6) -> mult3/1
  b_debus/2(out7) -> mult2/2
  a_debus/2(out7) -> mult2/1
  b_debus/1(msb_out8) -> mult1/2
  a_debus/1(msb_out8) -> mult1/1
  repb/1(out) -> b_debus/1(bus_in)
  repa/1(out) -> a_debus/1(bus_in)
  b/1 -> repb/1(in)
  a/1 -> repa/1(in)

== system r2_deng_tvg_rev1_13/control ==
  sim_1 : Inport
  sim_2 : Inport  Port=2
  sim_3 : Inport  Port=3
  sim_4 : Inport  Port=4
  sim_5 : Inport  Port=5
  sim_6 : Inport  Port=6
  sim_7 : Inport  Port=7
  sim_8 : Inport  Port=8
  sim_9 : Inport  Port=9
  convert1_{1..9} (9 alike) : DataTypeConversion  OutDataTypeStr=fixdt('ufix1_En0')  LockScale=on
  convert2_{1..9} (9 alike) : DataTypeConversion  OutDataTypeStr=fixdt('ufix1_En0')  ConvertRealWorld=Stored Integer (SI)  LockScale=on
  gain_1 : Gain  Gain=256
  gain_2 : Gain  Gain=128
  gain_3 : Gain  Gain=64
  gain_4 : Gain  Gain=32
  gain_5 : Gain  Gain=16
  gain_6 : Gain  Gain=8
  gain_7 : Gain  Gain=4
  gain_8 : Gain  Gain=2
  gain_9 : Gain
  io_delay : xbsIndex_r4/Delay  rst=off  infoeditControl=Selection of Reset will increase slice count due to use of real FFs and instead of SRLs  en=off  latency=1  dbl_ovrd=off  reg_retiming=on  block_type=delay
  r2_deng_tvg_rev1_13_control_user_data_out : xbsIndex_r4/Gateway In  gui_display_data_type=Fixed-point  arith_type=Unsigned  n_bits=32  bin_pt=0  preci_type=Single  exp_width=8  frac_width=24  quantization="Round  (unbiased: +/- Inf)"  overflow=Saturate  period=1  dbl_ovrd=off  timing_constraint=None  locs_specified=off  LOCs={}  UseAsADC=off  ADCChannel='1'  inherit_from_input=off  hdl_port=on  block_type=gatewayin
  reint2 : xbsIndex_r4/Reinterpret  force_arith_type=on  arith_type=Unsigned  force_bin_pt=on  bin_pt=0  block_type=reinterpret
  reint3 : xbsIndex_r4/Reinterpret  force_arith_type=on  arith_type=Unsigned  force_bin_pt=on  bin_pt=0  block_type=reinterpret
  sim_add : Sum  Inputs=+++++++++  OutDataTypeStr=uint32
  slice_clr_status : xbsIndex_r4/Slice  nbits=1  boolean_output=on  mode=Lower Bit Location + Width  bit1=0  base1=MSB of Input  bit0=5  base0=LSB of Input  dbl_ovrd=off  block_type=slice
  slice_gbe_rst : xbsIndex_r4/Slice  nbits=1  boolean_output=on  mode=Lower Bit Location + Width  bit1=0  base1=MSB of Input  bit0=4  base0=LSB of Input  dbl_ovrd=off  block_type=slice
  slice_gbe_txen : xbsIndex_r4/Slice  nbits=1  boolean_output=on  mode=Lower Bit Location + Width  bit1=0  base1=MSB of Input  bit0=3  base0=LSB of Input  dbl_ovrd=off  block_type=slice
  slice_load_tick_offset : xbsIndex_r4/Slice  nbits=1  boolean_output=on  mode=Lower Bit Location + Width  bit1=0  base1=MSB of Input  bit0=0  base0=LSB of Input  dbl_ovrd=off  block_type=slice
  slice_mrst : xbsIndex_r4/Slice  nbits=1  boolean_output=on  mode=Lower Bit Location + Width  bit1=0  base1=MSB of Input  bit0=1  base0=LSB of Input  dbl_ovrd=off  block_type=slice
  slice_msync : xbsIndex_r4/Slice  nbits=1  boolean_output=on  mode=Lower Bit Location + Width  bit1=0  base1=MSB of Input  bit0=2  base0=LSB of Input  dbl_ovrd=off  block_type=slice
  slice_tvg_select0 : xbsIndex_r4/Slice  nbits=1  boolean_output=off  mode=Lower Bit Location + Width  bit1=0  base1=MSB of Input  bit0=7  base0=LSB of Input  dbl_ovrd=off  block_type=slice
  slice_tvg_select1 : xbsIndex_r4/Slice  nbits=1  boolean_output=off  mode=Lower Bit Location + Width  bit1=0  base1=MSB of Input  bit0=6  base0=LSB of Input  dbl_ovrd=off  block_type=slice
  slice_up_cnt_rst : xbsIndex_r4/Slice  nbits=1  boolean_output=on  mode=Lower Bit Location + Width  bit1=0  base1=MSB of Input  bit0=8  base0=LSB of Input  dbl_ovrd=off  block_type=slice
  in_up_cnt_rst : Outport
  in_tvg_select0 : Outport  Port=2
  in_tvg_select1 : Outport  Port=3
  in_clr_status : Outport  Port=4
  in_gbe_rst : Outport  Port=5
  in_gbe_txen : Outport  Port=6
  in_msync : Outport  Port=7
  in_mrst : Outport  Port=8
  in_load_tick_offset : Outport  Port=9
  wires:
  r2_deng_tvg_rev1_13_control_user_data_out/1 -> io_delay/1
  sim_add/1 -> r2_deng_tvg_rev1_13_control_user_data_out/1
  sim_1/1 -> convert1_1/1
  convert1_1/1 -> convert2_1/1
  convert2_1/1 -> gain_1/1
  gain_1/1 -> sim_add/1
  io_delay/1 -> slice_up_cnt_rst/1, slice_tvg_select0/1, slice_tvg_select1/1, slice_clr_status/1, slice_gbe_rst/1, slice_gbe_txen/1, slice_msync/1, slice_mrst/1, slice_load_tick_offset/1
  slice_up_cnt_rst/1 -> in_up_cnt_rst/1
  sim_2/1 -> convert1_2/1
  convert1_2/1 -> convert2_2/1
  convert2_2/1 -> gain_2/1
  gain_2/1 -> sim_add/2
  slice_tvg_select0/1 -> reint2/1
  reint2/1 -> in_tvg_select0/1
  sim_3/1 -> convert1_3/1
  convert1_3/1 -> convert2_3/1
  convert2_3/1 -> gain_3/1
  gain_3/1 -> sim_add/3
  slice_tvg_select1/1 -> reint3/1
  reint3/1 -> in_tvg_select1/1
  sim_4/1 -> convert1_4/1
  convert1_4/1 -> convert2_4/1
  convert2_4/1 -> gain_4/1
  gain_4/1 -> sim_add/4
  slice_clr_status/1 -> in_clr_status/1
  sim_5/1 -> convert1_5/1
  convert1_5/1 -> convert2_5/1
  convert2_5/1 -> gain_5/1
  gain_5/1 -> sim_add/5
  slice_gbe_rst/1 -> in_gbe_rst/1
  sim_6/1 -> convert1_6/1
  convert1_6/1 -> convert2_6/1
  convert2_6/1 -> gain_6/1
  gain_6/1 -> sim_add/6
  slice_gbe_txen/1 -> in_gbe_txen/1
  sim_7/1 -> convert1_7/1
  convert1_7/1 -> convert2_7/1
  convert2_7/1 -> gain_7/1
  gain_7/1 -> sim_add/7
  slice_msync/1 -> in_msync/1
  sim_8/1 -> convert1_8/1
  convert1_8/1 -> convert2_8/1
  convert2_8/1 -> gain_8/1
  gain_8/1 -> sim_add/8
  slice_mrst/1 -> in_mrst/1
  sim_9/1 -> convert1_9/1
  convert1_9/1 -> convert2_9/1
  convert2_9/1 -> gain_9/1
  gain_9/1 -> sim_add/9
  slice_load_tick_offset/1 -> in_load_tick_offset/1

== system r2_deng_tvg_rev1_13/control_output ==
  sim_1 : Inport
  sim_2 : Inport  Port=2
  sim_3 : Inport  Port=3
  sim_4 : Inport  Port=4
  convert1_1 : DataTypeConversion  OutDataTypeStr=fixdt('ufix1_En0')  LockScale=on
  convert1_2 : DataTypeConversion  OutDataTypeStr=fixdt('ufix1_En0')  LockScale=on
  convert1_3 : DataTypeConversion  OutDataTypeStr=fixdt('ufix3_En0')  LockScale=on
  convert1_4 : DataTypeConversion  OutDataTypeStr=fixdt('ufix3_En0')  LockScale=on
  convert2_1 : DataTypeConversion  OutDataTypeStr=fixdt('ufix1_En0')  ConvertRealWorld=Stored Integer (SI)  LockScale=on
  convert2_2 : DataTypeConversion  OutDataTypeStr=fixdt('ufix1_En0')  ConvertRealWorld=Stored Integer (SI)  LockScale=on
  convert2_3 : DataTypeConversion  OutDataTypeStr=fixdt('ufix3_En0')  ConvertRealWorld=Stored Integer (SI)  LockScale=on
  convert2_4 : DataTypeConversion  OutDataTypeStr=fixdt('ufix3_En0')  ConvertRealWorld=Stored Integer (SI)  LockScale=on
  gain_1 : Gain  Gain=128
  gain_2 : Gain  Gain=64
  gain_3 : Gain  Gain=8
  gain_4 : Gain
  io_delay : xbsIndex_r4/Delay  rst=off  infoeditControl=Selection of Reset will increase slice count due to use of real FFs and instead of SRLs  en=off  latency=1  dbl_ovrd=off  reg_retiming=on  block_type=delay
  r2_deng_tvg_rev1_13_control_output_user_data_out : xbsIndex_r4/Gateway In  gui_display_data_type=Fixed-point  arith_type=Unsigned  n_bits=32  bin_pt=0  preci_type=Single  exp_width=8  frac_width=24  quantization="Round  (unbiased: +/- Inf)"  overflow=Saturate  period=1  dbl_ovrd=off  timing_constraint=None  locs_specified=off  LOCs={}  UseAsADC=off  ADCChannel='1'  inherit_from_input=off  hdl_port=on  block_type=gatewayin
  reint3 : xbsIndex_r4/Reinterpret  force_arith_type=on  arith_type=Unsigned  force_bin_pt=on  bin_pt=0  block_type=reinterpret
  reint4 : xbsIndex_r4/Reinterpret  force_arith_type=on  arith_type=Unsigned  force_bin_pt=on  bin_pt=0  block_type=reinterpret
  sim_add : Sum  Inputs=++++  OutDataTypeStr=uint32
  slice_load_en_time : xbsIndex_r4/Slice  nbits=1  boolean_output=on  mode=Lower Bit Location + Width  bit1=0  base1=MSB of Input  bit0=7  base0=LSB of Input  dbl_ovrd=off  block_type=slice
  slice_reset_en_time : xbsIndex_r4/Slice  nbits=1  boolean_output=on  mode=Lower Bit Location + Width  bit1=0  base1=MSB of Input  bit0=6  base0=LSB of Input  dbl_ovrd=off  block_type=slice
  slice_sample_end : xbsIndex_r4/Slice  nbits=3  boolean_output=off  mode=Lower Bit Location + Width  bit1=0  base1=MSB of Input  bit0=0  base0=LSB of Input  dbl_ovrd=off  block_type=slice
  slice_sample_start : xbsIndex_r4/Slice  nbits=3  boolean_output=off  mode=Lower Bit Location + Width  bit1=0  base1=MSB of Input  bit0=3  base0=LSB of Input  dbl_ovrd=off  block_type=slice
  in_load_en_time : Outport
  in_reset_en_time : Outport  Port=2
  in_sample_start : Outport  Port=3
  in_sample_end : Outport  Port=4
  wires:
  r2_deng_tvg_rev1_13_control_output_user_data_out/1 -> io_delay/1
  sim_add/1 -> r2_deng_tvg_rev1_13_control_output_user_data_out/1
  sim_1/1 -> convert1_1/1
  convert1_1/1 -> convert2_1/1
  convert2_1/1 -> gain_1/1
  gain_1/1 -> sim_add/1
  io_delay/1 -> slice_load_en_time/1, slice_reset_en_time/1, slice_sample_start/1, slice_sample_end/1
  slice_load_en_time/1 -> in_load_en_time/1
  sim_2/1 -> convert1_2/1
  convert1_2/1 -> convert2_2/1
  convert2_2/1 -> gain_2/1
  gain_2/1 -> sim_add/2
  slice_reset_en_time/1 -> in_reset_en_time/1
  sim_3/1 -> convert1_3/1
  convert1_3/1 -> convert2_3/1
  convert2_3/1 -> gain_3/1
  gain_3/1 -> sim_add/3
  slice_sample_start/1 -> reint3/1
  reint3/1 -> in_sample_start/1
  sim_4/1 -> convert1_4/1
  convert1_4/1 -> convert2_4/1
  convert2_4/1 -> gain_4/1
  gain_4/1 -> sim_add/4
  slice_sample_end/1 -> reint4/1
  reint4/1 -> in_sample_end/1
